simulink model "S32K39_FaultLogic_NXP_Codegen_Harness"  (R2024a)
settings: Solver=FixedStepAuto  StartTime=0.0  StopTime=15  FixedStep=1  RelTol=1e-3
settings Model: DataDictionary=S32K39_FaultLogic_NXP_Codegen.sldd  CodeVerificationMode=processor-in-the-loop (pil)  PacingRate=0.100000  Creator=nxf64875  LastModifiedBy=nxf64875
settings DataIOCC: SaveOutput=off  SaveTime=off
settings OptimizationCC: DefaultUnderspecifiedDataType=single  EnhancedBackFolding=on  PassReuseOutputArgsAs=Individual arguments  ZeroExternalMemoryAtStartup=off  ZeroInternalMemoryAtStartup=off  MaxStackSize=64  OptimizeBlockOrder=speed  DifferentSizesBufferReuse=on  OptimizationCustomize=off  EfficientTunableParamExpr=on
settings DebuggingCC: SigSpecEnsureSampleTimeMsg=none  ParameterTunabilityLossMsg=error
settings HardwareCC: ProdBitPerPointer=32  ProdBitPerSizeT=32  ProdBitPerPtrDiffT=32  ProdLargestAtomicInteger=Long  ProdLargestAtomicFloat=Double  ProdWordSize=32  ProdHWDeviceType=ARM Compatible->ARM Cortex
settings ModelReferenceCC: ModelReferenceNumInstancesAllowed=Single  PropagateSignalLabelsOutOfModel=off
settings SFSimCC: MATLABDynamicMemAlloc=off
settings RTWCC: Description=Embedded Coder  SystemTargetFile=ert.tlc  HardwareBoard=NXP S32K3xx  TemplateMakefile=ert_default_tmf  Toolchain=S32DS GCC  BuildConfiguration=Faster Runs  PortableWordSizes=on  CodeExecutionProfiling=on  CodeProfilingInstrumentation=coarse
settings CodeAppCC: ForceParamTrailComments=on  IgnoreCustomStorageClasses=off  OperatorAnnotations=on  SimulinkDataObjDesc=on  SFDataObjDesc=on  InsertBlockDesc=on
settings ERTTargetCC: ExtModeTransport=1  ExtModeMexFile=ext_serial_win32_comm  ERTSrcFileBannerTemplate=mbd_s32k3_ert_code_template.cgt  ERTHdrFileBannerTemplate=mbd_s32k3_ert_code_template.cgt  ERTDataSrcFileTemplate=mbd_s32k3_ert_code_template.cgt  ERTDataHdrFileTemplate=mbd_s32k3_ert_code_template.cgt

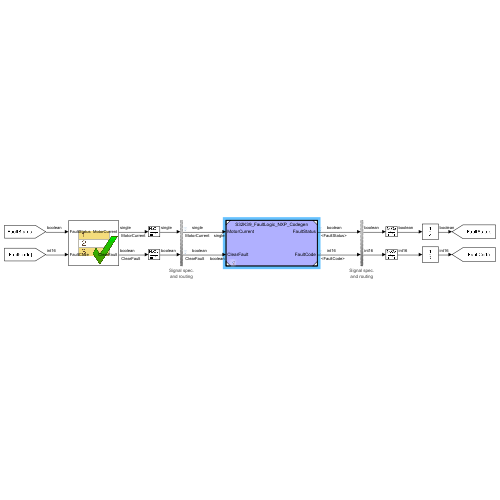
[thumbnail: Simulink's stored preview of the top-level diagram]
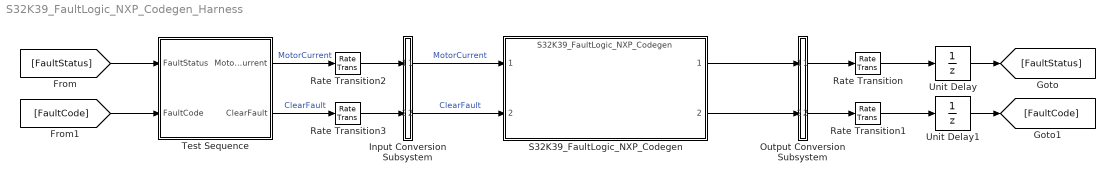
== system S32K39_FaultLogic_NXP_Codegen_Harness ==
  Input Conversion Subsystem : Subsystem  Tag=__SLT_ICS__  Description=|
      | Signal spec.
      | and routing
      settings: AttributesFormatString=%<Description>
  Output Conversion Subsystem : Subsystem  Tag=__SLT_OCS__  Description=|
      | Signal spec.
      | and routing
      settings: AttributesFormatString=%<Description>
  Rate Transition{,1..3} (4 alike) : RateTransition  OutPortSampleTimeOpt=Inherit
  S32K39_FaultLogic_NXP_Codegen : ModelReference  ModelNameDialog=S32K39_FaultLogic_NXP_Codegen  SimulationMode=Normal  ModelReferenceVersion=1.27
  Test Sequence : Test Sequence  TreatAsAtomicUnit=on
  Unit Delay : UnitDelay  SampleTime=-1  HasFrameUpgradeWarning=on
  Unit Delay1 : UnitDelay  SampleTime=-1  HasFrameUpgradeWarning=on
  wires:
  S32K39_FaultLogic_NXP_Codegen/1 -> Output Conversion Subsystem/1(Inport_1)
  S32K39_FaultLogic_NXP_Codegen/2 -> Output Conversion Subsystem/2(Inport_2)
  Output Conversion Subsystem/2(Outport_2) -> Rate Transition1/1
  [FaultStatus] -> Test Sequence/1(FaultStatus)
  [FaultCode] -> Test Sequence/2(FaultCode)
  Test Sequence/1(MotorCurrent) -> Rate Transition2/1  "MotorCurrent"
  Test Sequence/2(ClearFault) -> Rate Transition3/1  "ClearFault"
  Input Conversion Subsystem/1(Outport_1) -> S32K39_FaultLogic_NXP_Codegen/1  "MotorCurrent"
  Input Conversion Subsystem/2(Outport_2) -> S32K39_FaultLogic_NXP_Codegen/2  "ClearFault"
  Output Conversion Subsystem/1(Outport_1) -> Rate Transition/1
  Unit Delay/1 -> [FaultStatus]
  Unit Delay1/1 -> [FaultCode]
  Rate Transition/1 -> Unit Delay/1
  Rate Transition1/1 -> Unit Delay1/1
  Rate Transition2/1 -> Input Conversion Subsystem/1(Inport_1)
  Rate Transition3/1 -> Input Conversion Subsystem/2(Inport_2)

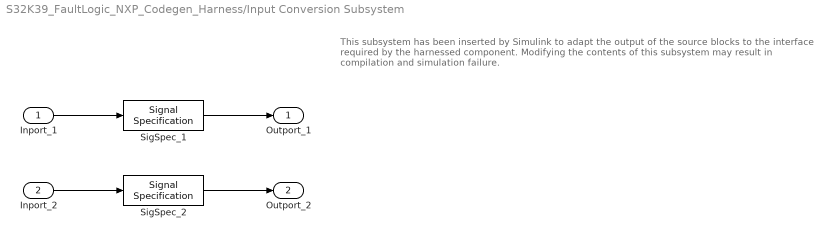
== system S32K39_FaultLogic_NXP_Codegen_Harness/Input Conversion Subsystem ==
  note: This subsystem has been inserted by Simulink to adapt the output of the source blocks to the interface required by the harnessed component.
      |  Modifying the contents of this subsystem may result in compilation and simulation failure.
  Inport_1 : Inport
  Inport_2 : Inport  Port=2
  SigSpec_1 : SignalSpecification  OutDataTypeStr=single  Dimensions=[1]  SampleTime=[0, 0]
  SigSpec_2 : SignalSpecification  OutDataTypeStr=boolean  Dimensions=[1]  SampleTime=[0, 0]
  Outport_1 : Outport
  Outport_2 : Outport  Port=2
  wires:
  SigSpec_1/1 -> Outport_1/1
  Inport_1/1 -> SigSpec_1/1
  SigSpec_2/1 -> Outport_2/1
  Inport_2/1 -> SigSpec_2/1

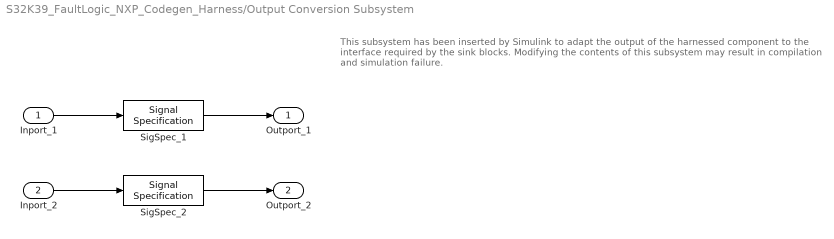
== system S32K39_FaultLogic_NXP_Codegen_Harness/Output Conversion Subsystem ==
  note: This subsystem has been inserted by Simulink to adapt the output of the harnessed component to the interface required by the sink blocks.
      |  Modifying the contents of this subsystem may result in compilation and simulation failure.
  Inport_1 : Inport
  Inport_2 : Inport  Port=2
  SigSpec_1 : SignalSpecification  OutDataTypeStr=boolean  Dimensions=[1]
  SigSpec_2 : SignalSpecification  OutDataTypeStr=int16  Dimensions=[1]
  Outport_1 : Outport
  Outport_2 : Outport  Port=2
  wires:
  Inport_1/1 -> SigSpec_1/1
  SigSpec_1/1 -> Outport_1/1
  Inport_2/1 -> SigSpec_2/1
  SigSpec_2/1 -> Outport_2/1

== stateflow chart S32K39_FaultLogic_NXP_Codegen_Harness/Test Sequence ==
  state OverLoadNoFault
    state Init
      MotorCurrent = single(3.0);
      ClearFault = false;
    state TriggerOverLoad
      MotorCurrent = single(5.8);
    state CheckOverLoad
      verify(hasChangedTo(FaultCode, int16(1)), 'Req1:FaultCode','MotorCurrent is %d and FaultCode is %d',MotorCurrent,FaultCode)
    state OverLoadStaysActive
    state UnderOverLoadThreshold
      MotorCurrent = single(1.2);
    state CheckOverLoadCleared
      verify(FaultCode == int16(0), 'Req1:FaultCode','MotorCurrent is %d and FaultCode is %d',MotorCurrent,FaultCode)
      verify(FaultStatus == false, 'Req1:FaultStatus','MotorCurrent is %d and FaultStatus is %d',MotorCurrent,FaultStatus)
    state LastStep
    (default) -> OverLoadNoFault.Init
    OverLoadNoFault.Init -> OverLoadNoFault.TriggerOverLoad : [
        | after(1,sec)
        | ]
    OverLoadNoFault.TriggerOverLoad -> OverLoadNoFault.CheckOverLoad : [
        | et(sec)>0.5
        | ]
    OverLoadNoFault.CheckOverLoad -> OverLoadNoFault.OverLoadStaysActive
    OverLoadNoFault.OverLoadStaysActive -> UnderOverLoadThreshold : [
        | after(2,sec)
        | ]
    UnderOverLoadThreshold -> CheckOverLoadCleared : [
        | after(1,sec)
        | ]
    CheckOverLoadCleared -> OverLoadNoFault.LastStep
  state OverLoadFault
    state Init
      MotorCurrent = single(3);
      ClearFault = false;
    state TriggerOverLoad
      MotorCurrent = single(5.6);
    state CheckOverLoad
      verify(hasChangedTo(FaultCode, int16(1)), 'Req2:FaultCode','MotorCurrent is %d and FaultCode is %d',MotorCurrent,FaultCode)
    state OverLoadActiveMoreThan5Sec
    state CheckOverLoadFault
      verify(hasChangedTo(FaultCode, int16(2)), 'Req2:FaultCode','MotorCurrent is %d and FaultCode is %d',MotorCurrent,FaultCode)
      verify(hasChangedTo(FaultStatus, true), 'Req2:FaultStatus','MotorCurrent is %d and FaultStatus is %d',MotorCurrent,FaultStatus)
    state ClearFault
      MotorCurrent = single(2);
      ClearFault = true;
    state LastStep
    (default) -> OverLoadFault.Init
    OverLoadFault.Init -> OverLoadFault.TriggerOverLoad : [
        | after(1, sec)
        | ]
    OverLoadFault.TriggerOverLoad -> OverLoadFault.CheckOverLoad : [
        | et(sec)>0.5
        | ]
    OverLoadFault.CheckOverLoad -> OverLoadActiveMoreThan5Sec
    OverLoadActiveMoreThan5Sec -> CheckOverLoadFault : [
        | after(5,sec)
        | ]
    CheckOverLoadFault -> OverLoadFault.ClearFault
    OverLoadFault.ClearFault -> OverLoadFault.LastStep : [
        | et(sec)>7.001
        | ]
  state OverCurrentFault
    state Init
      MotorCurrent = single(8);
      ClearFault = false;
    state CheckOverCurrent
      verify(hasChangedTo(FaultCode, int16(3)), 'Req4:FaultCode','MotorCurrent is %d and FaultCode is %d',MotorCurrent,FaultCode)
      verify(hasChangedTo(FaultStatus, true), 'Req4:FaultStatus','MotorCurrent is %d and FaultStatus is %d',MotorCurrent,FaultStatus)
    state OverCurrentActive
    state ClearFault
      MotorCurrent = single(3.5);
      ClearFault = true;
    state LastStep
    (default) -> OverCurrentFault.Init
    OverCurrentFault.Init -> OverCurrentFault.CheckOverCurrent : [
        | after(2, sec)
        | ]
    OverCurrentFault.CheckOverCurrent -> OverCurrentFault.OverCurrentActive : [
        | true
        | ]
    OverCurrentFault.OverCurrentActive -> OverCurrentFault.ClearFault : [
        | after(2,sec)
        | ]
    OverCurrentFault.ClearFault -> OverCurrentFault.LastStep : [
        | after(1,sec)
        | ]
  state OverCurrentFromOverLoad
    state Init
      MotorCurrent = single(3.5);
      ClearFault = false;
    state TriggerOverLoad
      MotorCurrent = single(5.6);
    state CheckOverLoad
      verify(hasChangedTo(FaultCode, int16(1)), 'Req1:FaultCode','MotorCurrent is %d and FaultCode is %d',MotorCurrent,FaultCode)
    state OverLoadStaysActive
    state OverCurrent
      MotorCurrent = single(8.5);
    state CheckOverCurrent
      verify(hasChangedTo(FaultCode, int16(3)), 'Req4:FaultCode','MotorCurrent is %d and FaultCode is %d',MotorCurrent,FaultCode)
      verify(hasChangedTo(FaultStatus, true), 'Req4:FaultStatus','MotorCurrent is %d and FaultStatus is %d',MotorCurrent,FaultStatus)
    state OverCurrentActive
    state LastStep
    (default) -> OverCurrentFromOverLoad.Init
    OverCurrentFromOverLoad.Init -> OverCurrentFromOverLoad.TriggerOverLoad : [
        | after(1,sec)
        | ]
    OverCurrentFromOverLoad.TriggerOverLoad -> OverCurrentFromOverLoad.CheckOverLoad : [
        | after(1,sec)
        | ]
    OverCurrentFromOverLoad.CheckOverLoad -> OverCurrentFromOverLoad.OverLoadStaysActive : [
        | true
        | ]
    OverCurrentFromOverLoad.OverLoadStaysActive -> OverCurrent : [
        | after(2,sec)
        | ]
    OverCurrent -> OverCurrentFromOverLoad.CheckOverCurrent : [
        | after(1,sec)
        | ]
    OverCurrentFromOverLoad.CheckOverCurrent -> OverCurrentFromOverLoad.OverCurrentActive : [
        | true
        | ]
    OverCurrentFromOverLoad.OverCurrentActive -> OverCurrentFromOverLoad.LastStep : [
        | after(2,sec)
        | ]
  (default) -> OverLoadNoFault [order 1] : [Active_Scenario_Index == 1]
  (default) -> OverLoadFault [order 2] : [Active_Scenario_Index == 2]
  (default) -> OverCurrentFault [order 3] : [Active_Scenario_Index == 3]
  (default) -> OverCurrentFromOverLoad [order 4] : {assert(Active_Scenario_Index == 4,'The value of Scenario Parameter ''Active_Scenario_Index'' is not valid. Use the index of the scenario to specify it.')}
  data: FaultStatus input boolean size=1; FaultCode input int16 size=1; MotorCurrent output single size=1; ClearFault output boolean size=1; Active_Scenario_Index parameter =4
